simulink model "angular_position_transfer_fucntion"  (R2017b)
settings: Solver=VariableStepAuto  StartTime=0.0  StopTime=8  RelTol=1e-3
settings Model: Creator=sysad  LastModifiedBy=sysad

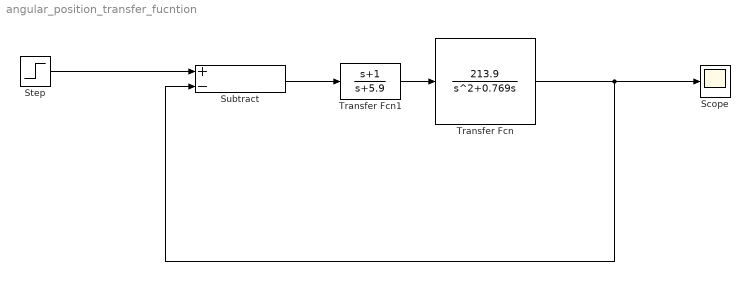
== system angular_position_transfer_fucntion ==
  Scope : Scope
  Step : Step  SampleTime=0.001
  Subtract : Sum  Inputs=+-
  Transfer Fcn : TransferFcn  Numerator=[213.9]  Denominator=[1 0.769 0]
  Transfer Fcn1 : TransferFcn  Numerator=[1 1]  Denominator=[1 5.9]
  wires:
  Step/1 -> Subtract/1
  Transfer Fcn/1 -> Subtract/2, Scope/1
  Subtract/1 -> Transfer Fcn1/1
  Transfer Fcn1/1 -> Transfer Fcn/1
